simulink model "NL_Before_PLA_fil"  (R2019b)
settings: Solver=VariableStepAuto  StartTime=0.0  StopTime=testtime  RelTol=1e-3
InitFcn:
  | NL_Before_PLA_Test_Parameters
StopFcn:
  | Verify_NL_Before_PLA_fil
values from neighbouring files (symbols this model uses):
  cf_factor = min(cfsat, 10^(cfslope*cf/1e3 + cfconst)) * 2.0    [NL_Before_PLA_Test_Parameters.m]
  Fs = 48e3    (= 48000)    [NL_Before_PLA_Test_Parameters.m]
  multFac = max(2.95*max(1.0,1.5-spont/100), 4.3-0.2*cf/1e3)    [NL_Before_PLA_Test_Parameters.m]
  spont = 100    [NL_Before_PLA_Test_Parameters.m]
libraries: hdlmdlgenlib x2, dspsrcs4 x2, simulink x1, fillib x1
settings Model: Creator=mblun  LastModifiedBy=t96f346
settings OptimizationCC: BlockReduction=off  ConditionallyExecuteInputs=off  DefaultParameterBehavior=Inlined
settings DebuggingCC: AlgebraicLoopMsg=error  InheritedTsInSrcMsg=none
settings HardwareCC: ProdBitPerPointer=32  ProdBitPerSizeT=32  ProdBitPerPtrDiffT=32  ProdLargestAtomicFloat=None  ProdIntDivRoundTo=Undefined  ProdEndianess=Unspecified  ProdWordSize=32  ProdHWDeviceType=ASIC/FPGA->ASIC/FPGA  TargetBitPerPointer=64  TargetBitPerSizeT=64  TargetBitPerPtrDiffT=64  TargetLongLongMode=on  TargetIntDivRoundTo=Zero  TargetEndianess=LittleEndian  TargetWordSize=64  TargetHWDeviceType=Custom Processor->MATLAB Host Computer  ProdEqTarget=off
settings SFSimCC: CustomCodeUndefinedFunction=UseInterfaceOnly

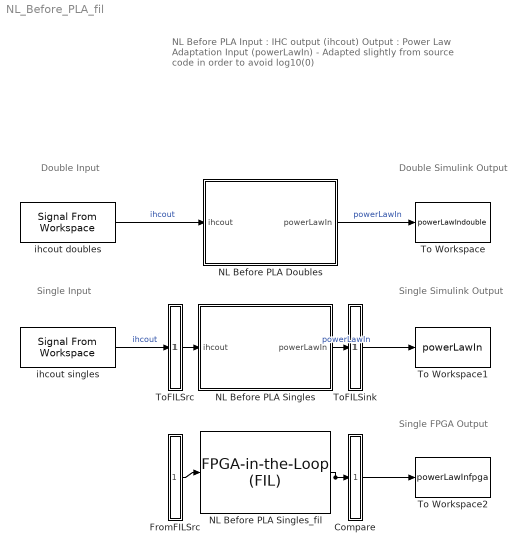
== system NL_Before_PLA_fil ==
  note: NL Before PLA
      |
      | Input : IHC output (ihcout)
      |
      | Output : Power Law Adaptation Input (powerLawIn)
      |
      | - Adapted slightly from source code in order to avoid log10(0)
  note: Double Simulink Output
  note: Single Simulink Output
  note: Single FPGA Output
  note: Double Input
  note: Single Input
  Compare : Subsystem
      mask Display: disp('')
  FromFILSrc : Subsystem
      mask Display: disp('')
  NL Before PLA Doubles : Subsystem
  NL Before PLA Singles : Subsystem
  NL Before PLA Singles_fil : fillib/FPGA-in-the-Loop (FIL)  ForceInterfaceUpdate=0.90579
      settings: SourceProductName=HDL Coder  SourceProductBaseCode=HD
  To Workspace : ToWorkspace  VariableName=powerLawIndouble  SampleTime=-1
      settings: Save2DSignal=2-D array (concatenate along first dimension)
  To Workspace1 : ToWorkspace  VariableName=powerLawIn  SampleTime=-1
      settings: Save2DSignal=2-D array (concatenate along first dimension)
  To Workspace2 : ToWorkspace  VariableName=powerLawInfpga  SampleTime=-1
      settings: Save2DSignal=2-D array (concatenate along first dimension)
  ToFILSink : Subsystem
      mask Display: disp('')
  ToFILSrc : Subsystem
      mask Display: disp('')
  "ihcout doubles " : dspsrcs4/Signal From Workspace  X=RxSignalDouble  Ts=1/Fs  nsamps=1  OutputAfterFinalValue=Setting to zero  ignoreOrWarnInputAndFrameLengths=off  OutputFrames=off
  ihcout singles : dspsrcs4/Signal From Workspace  X=RxSignal  Ts=1/Fs  nsamps=1  OutputAfterFinalValue=Setting to zero  ignoreOrWarnInputAndFrameLengths=off  OutputFrames=off
  wires:
  NL Before PLA Doubles/1(powerLawIn) -> To Workspace/1  "powerLawIn"
  "ihcout doubles "/1 -> NL Before PLA Doubles/1(ihcout)  "ihcout"
  ToFILSrc/1(out1) -> NL Before PLA Singles/1(ihcout)
  NL Before PLA Singles/1(powerLawIn) -> ToFILSink/1(in1)  "powerLawIn"
  ihcout singles/1 -> ToFILSrc/1(in1)  "ihcout"
  ToFILSink/1(out1) -> To Workspace1/1
  FromFILSrc/1(out1) -> NL Before PLA Singles_fil/1
  NL Before PLA Singles_fil/1 -> To Workspace2/1, Compare/1(in1)

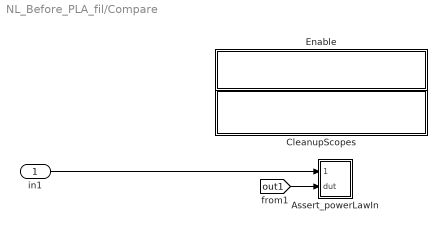
== system NL_Before_PLA_fil/Compare ==
  in1 : Inport
  Assert_powerLawIn : Subsystem  mask{ToleranceValue=1e-07}
  CleanupScopes : Subsystem
      settings: OpenFcn=|
      | blkName = gcb; %self block
      | idx = regexp(blkName, '/CleanupScopes$', 'once');
      | blkParent = blkName(1:idx-1);
      | blks=find_system(blkParent, 'LookUnderMasks', 'all','blocktype', 'Scope');
      | for itr = 1:length(blks)
      | 	 hScopeCfg = get_param(blks{itr},'ScopeConfiguration');
      | 	 hScopeCfg.Visible = ~ hScopeCfg.Visible;
      | end
      | drawnow;
      mask Display: fprintf(message('hdlcoder:cosim:vnl_dblclick').getString());
  Enable : Subsystem
      settings: OpenFcn=|
      | blkName = gcb;
      | idx = regexp(blkName, '/Enable$', 'once');
      | blkParent = blkName(1:idx-1);
      | blks=find_system(blkParent, 'LookUnderMasks', 'all','blocktype', 'Assertion');
      | e = get_param(blks{1}, 'Enabled');
      | if strcmp(e, 'on'), f= 'off';, else, f = 'on';, end
      | for ii=1:length(blks), set_param(blks{ii}, 'Enabled', f);, end
      | set_param(gcb, 'MaskDisplay',['fprintf(message(''hdlcoder:cosim:vnl_dblclick_assertions'',','''',upper(e),'''',').getString())']);
      mask Display: fprintf(message('hdlcoder:cosim:vnl_dblclick_assertions','OFF').getString());
  wires:
  in1/1 -> Assert_powerLawIn/1(cosim)
  [out1] -> Assert_powerLawIn/2(dut)

== system NL_Before_PLA_fil/FromFILSrc ==
  dtc1 : DataTypeConversion  OutDataTypeStr=single  SaturateOnIntegerOverflow=on  RndMeth=Zero
  out1 : Outport
  wires:
  [in1] -> dtc1/1
  dtc1/1 -> out1/1

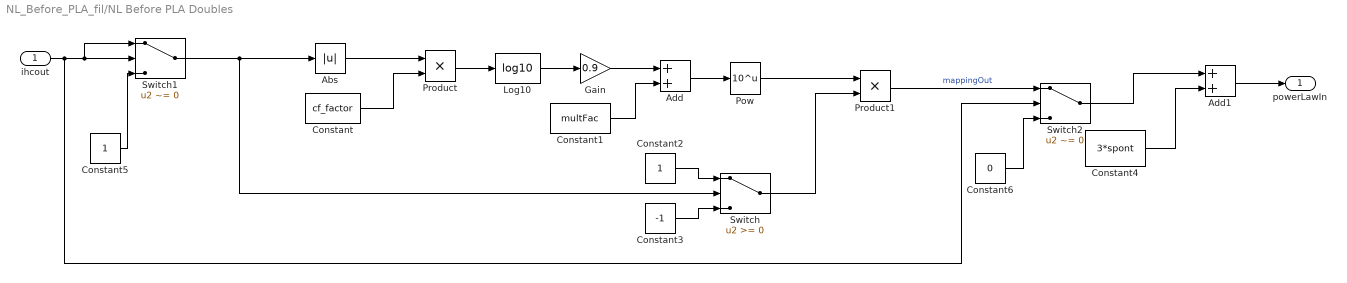
== system NL_Before_PLA_fil/NL Before PLA Doubles ==
  ihcout : Inport
  Abs : Abs
  Add : Sum
  Add1 : Sum
  Constant : Constant  Value=cf_factor  SampleTime=-1
  Constant1 : Constant  Value=multFac  SampleTime=-1
  Constant2 : Constant  SampleTime=-1
  Constant3 : Constant  Value=-1  SampleTime=-1
  Constant4 : Constant  Value=3*spont  SampleTime=-1
  Constant5 : Constant  SampleTime=-1
  Constant6 : Constant  Value=0  SampleTime=-1
  Gain : Gain  Gain=0.9
  Log10 : Math  Operator=log10  RndMeth=Zero  SaturateOnIntegerOverflow=on
  Pow : Math  Operator=10^u  RndMeth=Zero  SaturateOnIntegerOverflow=on
  Product : Product
  Product1 : Product
  Switch : Switch
  Switch1 : Switch  Criteria=u2 ~= 0  ZeroCross=off
  Switch2 : Switch  Criteria=u2 ~= 0  ZeroCross=off
  powerLawIn : Outport  VectorParamsAs1DForOutWhenUnconnected=off
  wires:
  Switch1/1 -> Switch/2, Abs/1
  Constant/1 -> Product/2
  Abs/1 -> Product/1
  Product/1 -> Log10/1
  Log10/1 -> Gain/1
  Gain/1 -> Add/1
  Constant1/1 -> Add/2
  Add/1 -> Pow/1
  Constant3/1 -> Switch/3
  Constant2/1 -> Switch/1
  Pow/1 -> Product1/1
  Switch/1 -> Product1/2
  Constant4/1 -> Add1/2
  Add1/1 -> powerLawIn/1
  ihcout/1 -> Switch2/2, Switch1/1, Switch1/2
  Constant6/1 -> Switch2/3
  Switch2/1 -> Add1/1
  Constant5/1 -> Switch1/3
  Product1/1 -> Switch2/1  "mappingOut"

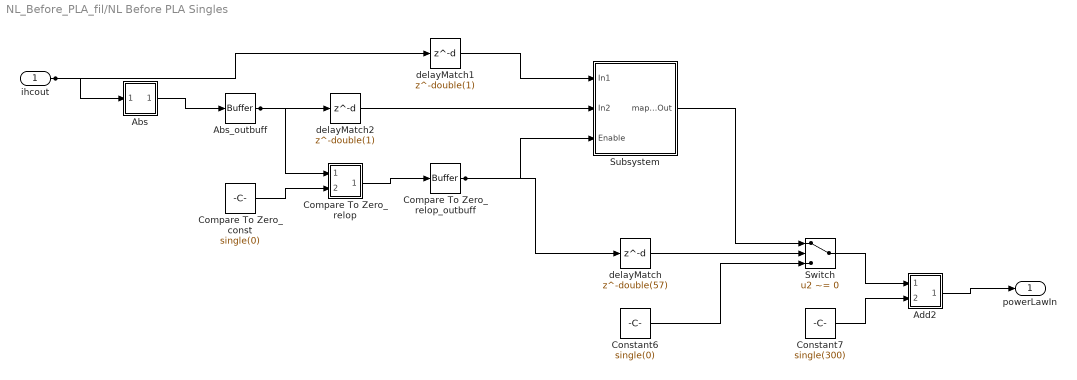
== system NL_Before_PLA_fil/NL Before PLA Singles ==
  ihcout : Inport  OutDataTypeStr=single  PortDimensions=1  SampleTime=2.08333333333333e-05
  Abs : Subsystem
      mask Display: disp('NFP\nabs');
  Abs_outbuff : hdlmdlgenlib/Buffer
      settings: SourceProductName=Simulink  SourceProductBaseCode=SL
  Add2 : Subsystem
      mask Display: disp('NFP\nadd');
  Compare To Zero_const : Constant  Value=single(0)  OutDataTypeStr=single  SampleTime=-1
  Compare To Zero_relop : Subsystem
      mask Display: disp('NFP\nrelop');
  Compare To Zero_relop_outbuff : hdlmdlgenlib/Buffer
      settings: SourceProductName=Simulink  SourceProductBaseCode=SL
  Constant6 : Constant  Value=single(0)  OutDataTypeStr=single  SampleTime=-1
  Constant7 : Constant  Value=single(300)  OutDataTypeStr=single  SampleTime=-1
  Subsystem : Subsystem
  Switch : Switch  Criteria=u2 ~= 0  Threshold=double(0)  OutDataTypeStr=single  SampleTime=2.08333333333333e-05
  delayMatch : Delay  DelayLength=double(57)  InitialCondition=0  SampleTime=2.08333333333333e-05
  delayMatch1 : Delay  DelayLength=double(1)  InitialCondition=0  SampleTime=2.08333333333333e-05
  delayMatch2 : Delay  DelayLength=double(1)  InitialCondition=0  SampleTime=2.08333333333333e-05
  powerLawIn : Outport  VectorParamsAs1DForOutWhenUnconnected=off
  wires:
  Abs_outbuff/1 -> Compare To Zero_relop/1(In1), delayMatch2/1
  ihcout/1 -> Abs/1(In1), delayMatch1/1
  Compare To Zero_relop/1(Out1) -> Compare To Zero_relop_outbuff/1
  Add2/1(Out1) -> powerLawIn/1
  Abs/1(Out1) -> Abs_outbuff/1
  Compare To Zero_relop_outbuff/1 -> Subsystem/3(Enable), delayMatch/1
  Compare To Zero_const/1 -> Compare To Zero_relop/2(In2)
  Switch/1 -> Add2/1(In1)
  Subsystem/1(mappingOut) -> Switch/1
  Constant7/1 -> Add2/2(In2)
  Constant6/1 -> Switch/3
  delayMatch/1 -> Switch/2
  delayMatch2/1 -> Subsystem/2(In2)
  delayMatch1/1 -> Subsystem/1(In1)

== system NL_Before_PLA_fil/ToFILSink ==
  in1 : Inport
  out1 : Outport
  tag scope: out1=global
  wires:
  in1/1 -> out1/1, [out1]

== system NL_Before_PLA_fil/ToFILSrc ==
  in1 : Inport
  out1 : Outport
  tag scope: in1=global
  wires:
  in1/1 -> out1/1, [in1]

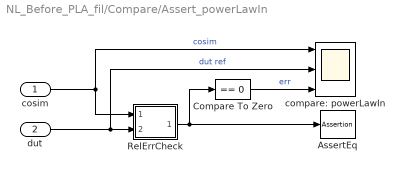
== system NL_Before_PLA_fil/Compare/Assert_powerLawIn ==
  cosim : Inport
  dut : Inport  Port=2
  AssertEq : Assertion  StopWhenAssertionFail=off
  Compare To Zero : simulink/Logic and Bit Operations/Compare To Zero  relop===  OutDataTypeStr=boolean
  RelErrCheck : Subsystem
  compare: powerLawIn : Scope  NumInputPorts=3
  wires:
  dut/1 -> compare: powerLawIn/2, RelErrCheck/2(In2)  "dut ref"
  cosim/1 -> compare: powerLawIn/1, RelErrCheck/1(In1)  "cosim"
  RelErrCheck/1(Out1) -> AssertEq/1, Compare To Zero/1
  Compare To Zero/1 -> compare: powerLawIn/3  "err"

== system NL_Before_PLA_fil/Compare/CleanupScopes ==

== system NL_Before_PLA_fil/Compare/Enable ==

== system NL_Before_PLA_fil/NL Before PLA Singles/Abs ==
  In1 : Inport
  Abs : Abs  SampleTime=2.08333333333333e-05  OutDataTypeStr=single
  Out1 : Outport
  wires:
  Abs/1 -> Out1/1
  In1/1 -> Abs/1

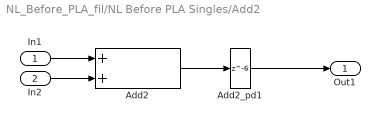
== system NL_Before_PLA_fil/NL Before PLA Singles/Add2 ==
  In1 : Inport
  In2 : Inport  Port=2
  Add2 : Sum  OutDataTypeStr=single  SampleTime=2.08333333333333e-05  SaturateOnIntegerOverflow=on  InputSameDT=on
  Add2_pd1 : Delay  DelayLength=6
  Out1 : Outport
  wires:
  Add2_pd1/1 -> Out1/1
  Add2/1 -> Add2_pd1/1
  In2/1 -> Add2/2
  In1/1 -> Add2/1

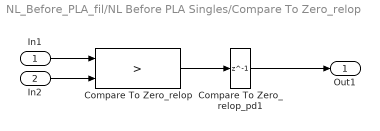
== system NL_Before_PLA_fil/NL Before PLA Singles/Compare To Zero_relop ==
  In1 : Inport
  In2 : Inport  Port=2
  Compare To Zero_relop : RelationalOperator  Operator=>  OutDataTypeStr=boolean  SampleTime=2.08333333333333e-05  RndMeth=Nearest  InputSameDT=on
  Compare To Zero_relop_pd1 : Delay  DelayLength=1
  Out1 : Outport
  wires:
  Compare To Zero_relop_pd1/1 -> Out1/1
  Compare To Zero_relop/1 -> Compare To Zero_relop_pd1/1
  In2/1 -> Compare To Zero_relop/2
  In1/1 -> Compare To Zero_relop/1

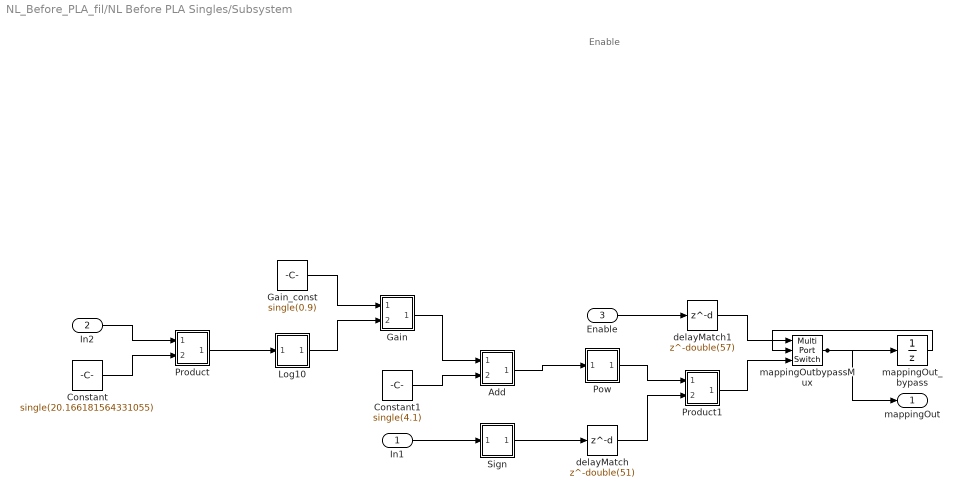
== system NL_Before_PLA_fil/NL Before PLA Singles/Subsystem ==
  note: Enable
  In1 : Inport  OutDataTypeStr=single  PortDimensions=1  SampleTime=2.08333333333333e-05
  In2 : Inport  Port=2  OutDataTypeStr=single  PortDimensions=1  SampleTime=2.08333333333333e-05
  Enable : Inport  Port=3  OutDataTypeStr=boolean  SampleTime=2.08333333333333e-05
  Add : Subsystem
      mask Display: disp('NFP\nadd');
  Constant : Constant  Value=single(20.166181564331055)  OutDataTypeStr=single  SampleTime=-1
  Constant1 : Constant  Value=single(4.1)  OutDataTypeStr=single  SampleTime=-1
  Gain : Subsystem
      mask Display: disp('NFP\nmul');
  Gain_const : Constant  Value=single(0.9)  OutDataTypeStr=single  SampleTime=-1
  Log10 : Subsystem
      mask Display: disp('NFP\nmath');
  Pow : Subsystem
      mask Display: disp('NFP\nmath');
  Product : Subsystem
      mask Display: disp('NFP\nmul');
  Product1 : Subsystem
      mask Display: disp('NFP\nmul');
  Sign : Subsystem
      mask Display: disp('NFP\nsignum');
  delayMatch : Delay  DelayLength=double(51)  InitialCondition=0
  delayMatch1 : Delay  DelayLength=double(57)  InitialCondition=0
  mappingOut_bypass : UnitDelay  SampleTime=2.08333333333333e-05
  mappingOutbypassMux : MultiPortSwitch  DataPortOrder=Zero-based contiguous  Inputs=2  zeroidx=on  OutDataTypeStr=single  SampleTime=2.08333333333333e-05
  mappingOut : Outport  InitialOutput=0
  wires:
  mappingOut_bypass/1 -> mappingOutbypassMux/2
  Enable/1 -> delayMatch1/1
  In2/1 -> Product/1(In1)
  In1/1 -> Sign/1(In1)
  mappingOutbypassMux/1 -> mappingOut_bypass/1, mappingOut/1
  Gain/1(Out1) -> Add/1(In1)
  Sign/1(Out1) -> delayMatch/1
  Product1/1(Out1) -> mappingOutbypassMux/3
  Product/1(Out1) -> Log10/1(In1)
  Pow/1(Out1) -> Product1/1(In1)
  Log10/1(Out1) -> Gain/2(In2)
  Add/1(Out1) -> Pow/1(In1)
  Gain_const/1 -> Gain/1(In1)
  delayMatch/1 -> Product1/2(In2)
  Constant1/1 -> Add/2(In2)
  Constant/1 -> Product/2(In2)
  delayMatch1/1 -> mappingOutbypassMux/1

== system NL_Before_PLA_fil/Compare/Assert_powerLawIn/RelErrCheck ==
  In1 : Inport
  In2 : Inport  Port=2
  "RelativeErrorCheck " : MATLAB Function  TreatAsAtomicUnit=on
  Out1 : Outport  VectorParamsAs1DForOutWhenUnconnected=off
  wires:
  In2/1 -> "RelativeErrorCheck "/2(R)
  In1/1 -> "RelativeErrorCheck "/1(P)
  "RelativeErrorCheck "/1(y) -> Out1/1

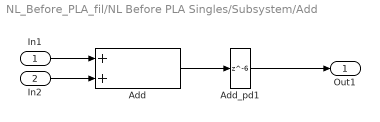
== system NL_Before_PLA_fil/NL Before PLA Singles/Subsystem/Add ==
  In1 : Inport
  In2 : Inport  Port=2
  Add : Sum  OutDataTypeStr=single  SampleTime=2.08333333333333e-05  SaturateOnIntegerOverflow=on  InputSameDT=on
  Add_pd1 : Delay  DelayLength=6
  Out1 : Outport
  wires:
  Add_pd1/1 -> Out1/1
  Add/1 -> Add_pd1/1
  In2/1 -> Add/2
  In1/1 -> Add/1

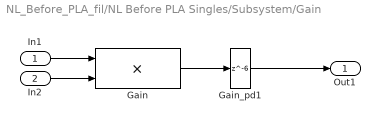
== system NL_Before_PLA_fil/NL Before PLA Singles/Subsystem/Gain ==
  In1 : Inport
  In2 : Inport  Port=2
  Gain : Product  Inputs=**  OutDataTypeStr=single  SampleTime=2.08333333333333e-05
  Gain_pd1 : Delay  DelayLength=6
  Out1 : Outport
  wires:
  Gain_pd1/1 -> Out1/1
  Gain/1 -> Gain_pd1/1
  In2/1 -> Gain/2
  In1/1 -> Gain/1

== system NL_Before_PLA_fil/NL Before PLA Singles/Subsystem/Log10 ==
  In1 : Inport
  Log10 : Math  Operator=log10  SampleTime=2.08333333333333e-05  SaturateOnIntegerOverflow=on
  Log10_pd1 : Delay  DelayLength=17
  Out1 : Outport
  wires:
  Log10_pd1/1 -> Out1/1
  Log10/1 -> Log10_pd1/1
  In1/1 -> Log10/1

== system NL_Before_PLA_fil/NL Before PLA Singles/Subsystem/Pow ==
  In1 : Inport
  Pow : Math  Operator=10^u  SampleTime=2.08333333333333e-05  SaturateOnIntegerOverflow=on
  Pow_pd1 : Delay  DelayLength=16
  Out1 : Outport
  wires:
  Pow_pd1/1 -> Out1/1
  Pow/1 -> Pow_pd1/1
  In1/1 -> Pow/1

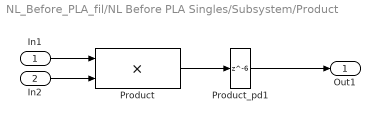
== system NL_Before_PLA_fil/NL Before PLA Singles/Subsystem/Product ==
  In1 : Inport
  In2 : Inport  Port=2
  Product : Product  Inputs=**  OutDataTypeStr=single  SampleTime=2.08333333333333e-05
  Product_pd1 : Delay  DelayLength=6
  Out1 : Outport
  wires:
  Product_pd1/1 -> Out1/1
  Product/1 -> Product_pd1/1
  In2/1 -> Product/2
  In1/1 -> Product/1

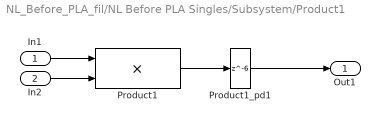
== system NL_Before_PLA_fil/NL Before PLA Singles/Subsystem/Product1 ==
  In1 : Inport
  In2 : Inport  Port=2
  Product1 : Product  Inputs=**  OutDataTypeStr=single  SampleTime=2.08333333333333e-05
  Product1_pd1 : Delay  DelayLength=6
  Out1 : Outport
  wires:
  Product1_pd1/1 -> Out1/1
  Product1/1 -> Product1_pd1/1
  In2/1 -> Product1/2
  In1/1 -> Product1/1

== system NL_Before_PLA_fil/NL Before PLA Singles/Subsystem/Sign ==
  In1 : Inport
  Sign : Signum  SampleTime=2.08333333333333e-05
  Out1 : Outport
  wires:
  Sign/1 -> Out1/1
  In1/1 -> Sign/1

== matlab function NL_Before_PLA_fil/Compare/Assert_powerLawIn/RelErrCheck/RelativeErrorCheck  ==
  data: P input; y output; R input; ToleranceValue parameter double
% Check if the relative error of R with respect to P is below
% ToleranceValue
% P, R are floating-point
function y = relErrCheck(P,R, ToleranceValue)
    tol = ToleranceValue;
    sz = numel(P);
    assert(sz == numel(R), 'Inputs P and R have different sizes.');
    y = false(1, sz);

    for ii=1:sz
        if (isnan(P(ii)) || isnan(R(ii)))
            if (isnan(P(ii)) && isnan(R(ii)))
                y(ii) = true;
            end
        elseif (isinf(P(ii)) || isinf(R(ii)))
            y(ii) = (P(ii) == R(ii));
        elseif (P(ii) == 0)
            y(ii) = (R(ii) == 0);
        else
            absdiff = abs(P(ii) - R(ii));
            relerr = absdiff/abs(P(ii));
            y(ii) = (relerr <= tol);
        end
    end
end
